simulink model "acc"  (R2018a)
settings: Solver=VariableStepAuto  StartTime=0.0  StopTime=300  FixedStep=0.02  RelTol=1e-3
values from neighbouring files (symbols this model uses):
  b_Ahead = 50    [ACC_DATA.m]    (also in CC_data.m)
  Ctr = 1.6    [ACC_DATA.m]
  F_aero = 1/(2*m_Follower) * Ro_A_Cd    (= 0.000326666666667)    [ACC_DATA.m]
  F_grav = g * sin(theta)    [ACC_DATA.m]
  F_res = Cr * g * cos(theta)    [ACC_DATA.m]
  Kb = 0.005    [ACC_DATA.m]
  Kc = 1    [ACC_DATA.m]
  m_Ahead = 1000    [ACC_DATA.m]    (also in CC_data.m)
  m_Follower = 1500    [ACC_DATA.m]
  r = 0.326    [ACC_DATA.m]
  Rf = 3.28    [ACC_DATA.m]
  Rtr = 1    [ACC_DATA.m]
  Tmax = 528.7 + 0.152*Ne - 0.0000217*Ne^2    (= 789.5)    [ACC_DATA.m]
undefined symbols (not defined in the file or in its folder): sigbuilder_block
libraries: simulink x7
settings Model: Creator=Talha Rao  LastModifiedBy=Talha Rao

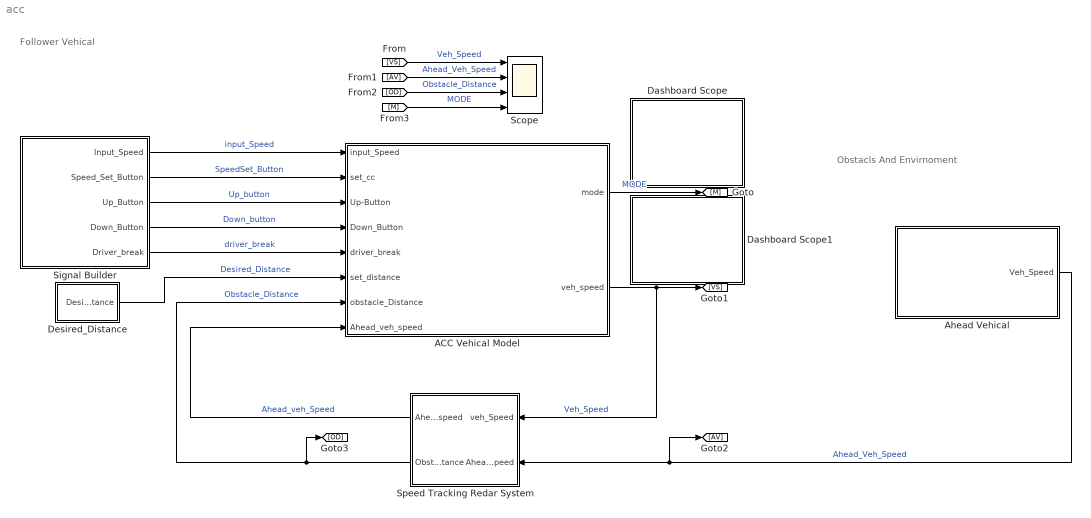
== system acc ==
  note: Follower Vehical
  note: Obstacls And Envirnoment
  ACC Vehical Model : Subsystem
      mask Display: image('C:\Users\Talha Rao\Pictures\carpaint_basic (2).png');
  Ahead Vehical : Subsystem
      mask Display: image('C:\Users\Talha Rao\Pictures\index2 (2).jpg');
  Dashboard Scope : Subsystem  DialogController=hmiCreateDDGDialog  IsWebBlock=on  mask(MWDashboardBlock){webBlockId=e8525703-5d25-447f-a1ea-0cd47b72d774, webBlockType=sdiscope, ShowInitialText=on, HMISrcModelName=acc}
      mask prompts: webBlockId "WebBlock Id"; webBlockType "WebBlock Type"; HMISrcModelName "Source Model"
      mask help: SimulinkHMI:dialogs:HMIScopeDialogDesc
      mask Help: helpview([docroot '/mapfiles/simulink.map'], 'hmi_scope')
      mask Display:
      | if strcmp(get_param(bdroot(gcb),'BlockDiagramType'), 'library')
      |     image([(matlabroot) '/toolbox/simulink/hmi/icons/DashboardScope.png']);
      | end
  Dashboard Scope1 : Subsystem  DialogController=hmiCreateDDGDialog  IsWebBlock=on  mask(MWDashboardBlock){webBlockId=d1b5fd32-8fa1-4132-bafa-763aef0d9398, webBlockType=sdiscope, ShowInitialText=on, HMISrcModelName=acc}
      mask prompts: webBlockId "WebBlock Id"; webBlockType "WebBlock Type"; HMISrcModelName "Source Model"
      mask help: SimulinkHMI:dialogs:HMIScopeDialogDesc
      mask Help: helpview([docroot '/mapfiles/simulink.map'], 'hmi_scope')
      mask Display:
      | if strcmp(get_param(bdroot(gcb),'BlockDiagramType'), 'library')
      |     image([(matlabroot) '/toolbox/simulink/hmi/icons/DashboardScope.png']);
      | end
  Desired_Distance : Subsystem  mask{Desired_Distance=25.0}
      mask DialogControl DescGroupVar Prompt: Set Desired Distance
      mask Display: image('C:\Users\Talha Rao\Pictures\070558928_iconm (2).jpeg');
  Scope : Scope  NumInputPorts=4
  Signal Builder : Subsystem  Tag=STV Subsys  LoadFcn=sigbuilder_block('load',[0 -132 1440 723.6 ]);  StartFcn=sigbuilder_block('start');  StopFcn=sigbuilder_block('stop');  ClipboardFcn=sigbuilder_block('clipboard');  mask(Sigbuilder block){tuvar=[0:10]}
      mask help: Simulink:masks:SigbuilderBlock_MD
      mask init:
      | if ~strcmp(get_param(bdroot(gcbh),'SimulationStatus'),'stopped') tuvar = sigbuilder_block('maskInit'); end
      settings: CopyFcn=sigbuilder_block('copy');  DeleteFcn=sigbuilder_block('delete');  ModelCloseFcn=sigbuilder_block('modelClose');  PreSaveFcn=sigbuilder_block('preSave');  PauseFcn=sigbuilder_block('pause');  ContinueFcn=sigbuilder_block('continue');  NameChangeFcn=sigbuilder_block('namechange');  OpenFcn=sigbuilder_block('open',[0 192 1152 560.25 ]);  CloseFcn=sigbuilder_block('close');
      mask Display: plot(0, 0, 100, 100,[2, 2, 32, 32, 2], [68, 8, 8, 68, 68],[32, 2], [38, 38], [32, 19, 2],[53, 60, 44], [32, 17, 17, 2],[16, 16, 31, 31]);txt = getActiveGroup(gcbh);text(2, 100, txt,'verticalAlignment', 'top');
  Speed Tracking Redar System : Subsystem
      mask Display: image('C:\Users\Talha Rao\Pictures\index3.png');
  wires:
  ACC Vehical Model/2(veh_speed) -> Speed Tracking Redar System/1(veh_Speed), [VS]  "Veh_Speed"
  Speed Tracking Redar System/2(Obstacle_Distance) -> [OD], ACC Vehical Model/7(obstacle_Distance)  "Obstacle_Distance"
  Ahead Vehical/1(Veh_Speed) -> [AV], Speed Tracking Redar System/2(Ahead_Veh_Speed)  "Ahead_Veh_Speed"
  Signal Builder/1(Input_Speed) -> ACC Vehical Model/1(input_Speed)  "input_Speed"
  Signal Builder/3(Up_Button) -> ACC Vehical Model/3(Up-Button)  "Up_button"
  Signal Builder/4(Down_Button) -> ACC Vehical Model/4(Down_Button)  "Down_button"
  Signal Builder/5(Driver_break) -> ACC Vehical Model/5(driver_break)  "driver_break"
  Desired_Distance/1(Desired_Distance) -> ACC Vehical Model/6("set_distance ")  "Desired_Distance"
  Speed Tracking Redar System/1(Ahead_veh_speed) -> ACC Vehical Model/8(Ahead_veh_speed)  "Ahead_veh_Speed"
  [VS] -> Scope/1  "Veh_Speed"
  [AV] -> Scope/2  "Ahead_Veh_Speed"
  [OD] -> Scope/3  "Obstacle_Distance"
  [M] -> Scope/4  "MODE"
  ACC Vehical Model/1(mode) -> [M]  "MODE"
  Signal Builder/2(Speed_Set_Button) -> ACC Vehical Model/2(set_cc)  "SpeedSet_Button"

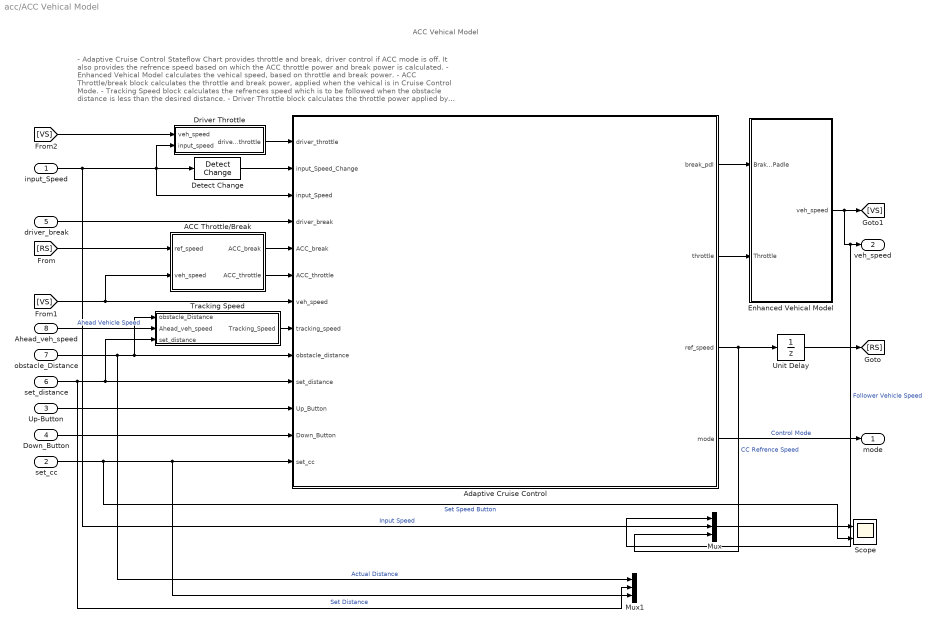
== system acc/ACC Vehical Model ==
  note: - Adaptive Cruise Control Stateflow Chart provides throttle and break, driver control if ACC mode is off. It also provides the refrence speed based on which the ACC throttle power and break power is calculated.
      | - Enhanced Vehical Model calculates the vehical speed, based on throttle and break power.
      | - ACC Throttle/break block calculates the throttle and break power, applied when the vehical is in Cruise Control Mode.
      | - Tracking Speed block calculates the refrences speed which is to be followed when the obstacle distance is less than the desired distance.
      | - Driver Throttle block calculates the throttle power applied by the driver
  note: ACC Vehical Model
  input_Speed : Inport
  set_cc : Inport  Port=2
  Up-Button : Inport  Port=3
  Down_Button : Inport  Port=4
  driver_break : Inport  Port=5
  "set_distance " : Inport  Port=6
  obstacle_Distance : Inport  Port=7
  Ahead_veh_speed : Inport  Port=8
  ACC Throttle/Break : Subsystem
  Adaptive Cruise Control : Stateflow chart  TreatAsAtomicUnit=on
  Detect Change : simulink/Logic and Bit Operations/Detect Change  vinit=0  OutDataTypeStr=boolean
  Driver Throttle : Subsystem
  Enhanced Vehical Model : Subsystem
  Mux : Mux  Inputs=3
  Mux1 : Mux  Inputs=3
  Scope : Scope  NumInputPorts=2
  Tracking Speed : Subsystem
  Unit Delay : UnitDelay  SampleTime=-1
  mode : Outport
  veh_speed : Outport  Port=2
  wires:
  Up-Button/1 -> Adaptive Cruise Control/11(Up_Button)
  Down_Button/1 -> Adaptive Cruise Control/12(Down_Button)
  Detect Change/1 -> Adaptive Cruise Control/2(input_Speed_Change)
  driver_break/1 -> Adaptive Cruise Control/4(driver_break)
  obstacle_Distance/1 -> Mux1/1, Adaptive Cruise Control/9(obstacle_distance), Tracking Speed/1(obstacle_Distance)  "Actual Distance"
  input_Speed/1 -> Mux/2, Adaptive Cruise Control/3(input_Speed), Detect Change/1, Driver Throttle/2(input_speed)  "Input Speed"
  "set_distance "/1 -> Mux1/2, Adaptive Cruise Control/10(set_distance), Tracking Speed/3(set_distance)  "Set Distance"
  ACC Throttle/Break/1(ACC_break) -> Adaptive Cruise Control/5(ACC_break)
  ACC Throttle/Break/2(ACC_throttle) -> Adaptive Cruise Control/6(ACC_throttle)
  [VS] -> Adaptive Cruise Control/7(veh_speed), ACC Throttle/Break/2(veh_speed)
  [RS] -> ACC Throttle/Break/1(ref_speed)
  Adaptive Cruise Control/1(break_pdl) -> Enhanced Vehical Model/1(Brake_Padle)
  Adaptive Cruise Control/2(throttle) -> Enhanced Vehical Model/2(Throttle)
  Enhanced Vehical Model/1(veh_speed) -> Mux/1, veh_speed/1, [VS]  "Follower Vehicle Speed"
  Unit Delay/1 -> [RS]
  Adaptive Cruise Control/4(mode) -> mode/1  "Control Mode"
  Tracking Speed/1(Tracking_Speed) -> Adaptive Cruise Control/8(tracking_speed)
  Ahead_veh_speed/1 -> Tracking Speed/2(Ahead_veh_speed)  "Ahead Vehicle Speed"
  Driver Throttle/1(driver_throttle) -> Adaptive Cruise Control/1(driver_throttle)
  [VS] -> Driver Throttle/1(veh_speed)
  Adaptive Cruise Control/3(ref_speed) -> Mux/3, Unit Delay/1  "CC Refrence Speed"
  set_cc/1 -> Scope/2, Mux1/3, Adaptive Cruise Control/13(set_cc)  "Set Speed Button"
  Mux/1 -> Scope/1

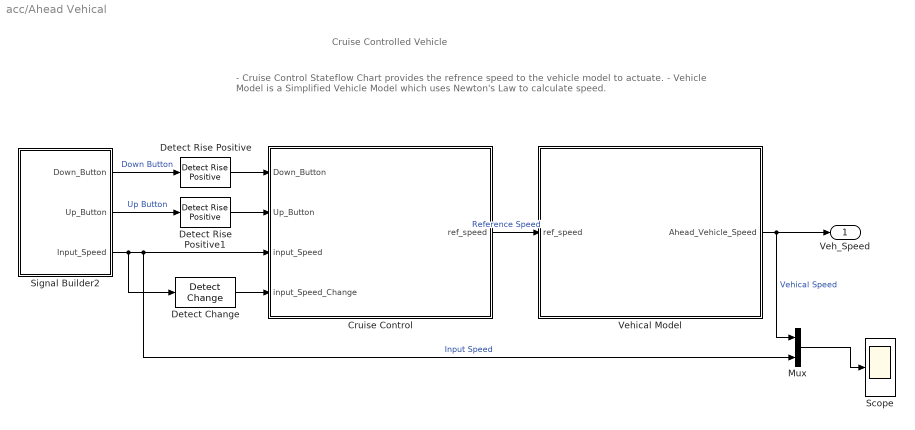
== system acc/Ahead Vehical ==
  note: - Cruise Control Stateflow Chart provides the refrence speed to the vehicle model to actuate.
      | - Vehicle Model is a Simplified Vehicle Model which uses Newton's Law to calculate speed.
  note: Cruise Controlled Vehicle
  Cruise Control : Stateflow chart  TreatAsAtomicUnit=on
  Detect Change : simulink/Logic and Bit Operations/Detect Change  vinit=0  OutDataTypeStr=boolean
  Detect Rise Positive : simulink/Logic and Bit Operations/Detect Rise Positive  vinit=0  OutDataTypeStr=boolean
  Detect Rise Positive1 : simulink/Logic and Bit Operations/Detect Rise Positive  vinit=0  OutDataTypeStr=boolean
  Mux : Mux  Inputs=2
  Scope : Scope
  Signal Builder2 : Subsystem  Tag=STV Subsys  LoadFcn=sigbuilder_block('load');  StartFcn=sigbuilder_block('start');  StopFcn=sigbuilder_block('stop');  ClipboardFcn=sigbuilder_block('clipboard');  mask(Sigbuilder block){tuvar=[0:10]}
      mask help: Simulink:masks:SigbuilderBlock_MD
      mask init:
      | if ~strcmp(get_param(bdroot(gcbh),'SimulationStatus'),'stopped') tuvar = sigbuilder_block('maskInit'); end
      settings: CopyFcn=sigbuilder_block('copy');  DeleteFcn=sigbuilder_block('delete');  ModelCloseFcn=sigbuilder_block('modelClose');  PreSaveFcn=sigbuilder_block('preSave');  PauseFcn=sigbuilder_block('pause');  ContinueFcn=sigbuilder_block('continue');  NameChangeFcn=sigbuilder_block('namechange');  OpenFcn=sigbuilder_block('open',[156 150.75 550.5 399.75 ]);  CloseFcn=sigbuilder_block('close');
      mask Display: plot(0, 0, 100, 100,[2, 2, 32, 32, 2], [68, 8, 8, 68, 68],[32, 2], [38, 38], [32, 19, 2],[53, 60, 44], [32, 17, 17, 2],[16, 16, 31, 31]);txt = getActiveGroup(gcbh);text(2, 100, txt,'verticalAlignment', 'top');
  Vehical Model : Subsystem
  Veh_Speed : Outport
  wires:
  Vehical Model/1(Ahead_Vehicle_Speed) -> Mux/1, Veh_Speed/1  "Vehical Speed"
  Detect Change/1 -> Cruise Control/4(input_Speed_Change)
  Cruise Control/1(ref_speed) -> Vehical Model/1(ref_speed)  "Reference Speed"
  Detect Rise Positive/1 -> Cruise Control/1(Down_Button)
  Signal Builder2/3(Input_Speed) -> Detect Change/1, Mux/2, Cruise Control/3(input_Speed)  "Input Speed"
  Signal Builder2/2(Up_Button) -> Detect Rise Positive1/1  "Up Button"
  Signal Builder2/1(Down_Button) -> Detect Rise Positive/1  "Down Button"
  Detect Rise Positive1/1 -> Cruise Control/2(Up_Button)
  Mux/1 -> Scope/1

== system acc/Dashboard Scope ==

== system acc/Dashboard Scope1 ==

== system acc/Desired_Distance ==
  Constant : Constant  Value=Desired_Distance
  Desired_Distance : Outport
  wires:
  Constant/1 -> Desired_Distance/1

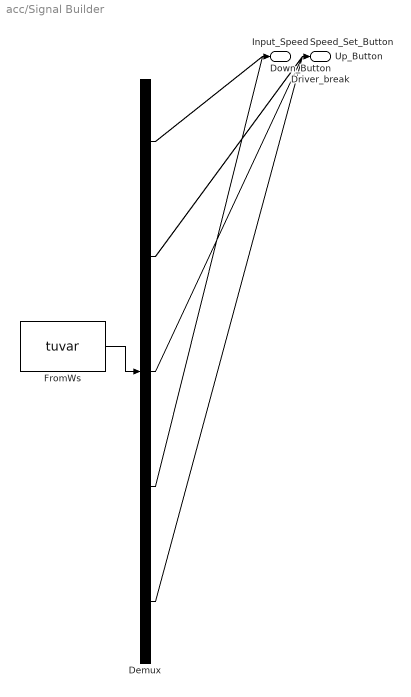
== system acc/Signal Builder ==
  Demux : Demux  Tag=STV Demux  Outputs=5
  FromWs : FromWorkspace  Tag=STV FromWs  VariableName=tuvar  SampleTime=0
      SigBuilderData=|
      | common.afterFinalStr = 'Extrapolate'
      | common.sampleTime = 0
      | dataSet.timeRange = [0 200]
      | dataSet.name = 'Group 1'
      | sbobj.Groups.Name = 'Group 1'
      | sbobj.Groups.Signals(1).Name = 'Input_Speed'
      | sbobj.Groups.Signals(1).XData = [0 12 30 42 43 200]
      | sbobj.Groups.Signals(1).YData = [0 0 112 112 0 0]
      | sbobj.Groups.Signals(2).Name = 'Speed_Set_Button'
      | sbobj.Groups.Signals(2).XData = [0 31 33 200]
      | sbobj.Groups.Signals(2).YData = [0 0 0 0]
      | sbobj.Groups.Signals(3).Name = 'Up_Button'
      | sbobj.Groups.Signals(3).XData = [0 1 200]
      | sbobj.Groups.Signals(3).YData = [0 0 0]
      | sbobj.Groups.Signals(4).Name = 'Down_Button'
      | sbobj.Groups.Signals(4).XData = [0 3 3.4 6 6.4 7 7.4 200]
      | sbobj.Groups.Signals(4).YData = [0 0 0 0 0 0 0 0]
      | sbobj.Groups.Signals(5).Name = 'Driver_break'
      | sbobj.Groups.Signals(5).XData = [0 200]
      | sbobj.Groups.Signals(5).YData = [0 0]
      | sbobj.Groups.TimeRange = [0 200]
  Input_Speed : Outport  Tag=STV Outport
  Speed_Set_Button : Outport  Tag=STV Outport  Port=2
  Up_Button : Outport  Tag=STV Outport  Port=3
  Down_Button : Outport  Tag=STV Outport  Port=4
  Driver_break : Outport  Tag=STV Outport  Port=5
  wires:
  FromWs/1 -> Demux/1
  Demux/1 -> Input_Speed/1
  Demux/2 -> Speed_Set_Button/1
  Demux/3 -> Up_Button/1
  Demux/4 -> Down_Button/1
  Demux/5 -> Driver_break/1

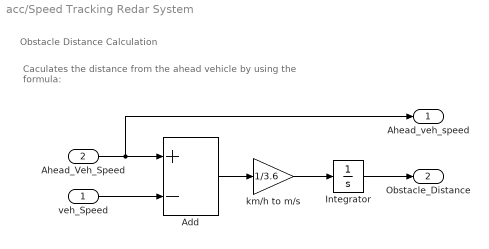
== system acc/Speed Tracking Redar System ==
  note: Caculates the distance from the ahead vehicle by using the formula:
  note: Obstacle Distance Calculation
  veh_Speed : Inport
  Ahead_Veh_Speed : Inport  Port=2
  Add : Sum  Inputs=+-
  Integrator : Integrator  InitialCondition=100
  km/h to m/s : Gain  Gain=1/3.6
  Ahead_veh_speed : Outport
  Obstacle_Distance : Outport  Port=2
  wires:
  Ahead_Veh_Speed/1 -> Ahead_veh_speed/1, Add/1
  veh_Speed/1 -> Add/2
  Add/1 -> km/h to m/s/1
  km/h to m/s/1 -> Integrator/1
  Integrator/1 -> Obstacle_Distance/1

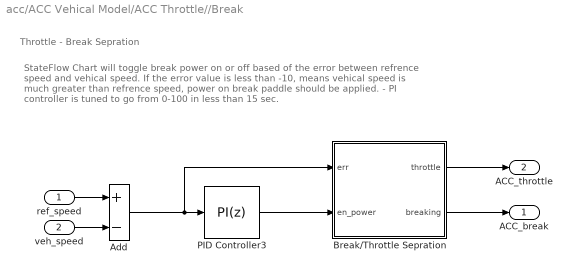
== system acc/ACC Vehical Model/ACC Throttle//Break ==
  note: StateFlow Chart will toggle break power on or off based of the error between refrence speed and
      | vehical speed. If the error value is less than -10, means vehical speed is much greater than refrence
      | speed, power on break paddle should be applied.
      |
      | - PI controller is tuned to go from 0-100 in less than 15 sec.
  note: Throttle - Break Sepration
  ref_speed : Inport
  veh_speed : Inport  Port=2
  Add : Sum  Inputs=+-
  Break/Throttle Sepration : Stateflow chart  TreatAsAtomicUnit=on
  PID Controller3 : simulink/Continuous/PID Controller  Controller=PI  TimeDomain=Discrete-time  SampleTime=0.02  IntegratorMethod=Trapezoidal  FilterMethod=Forward Euler  Form=Parallel  UseFilter=on  ControllerParametersSource=internal  P=5  I=0.5  D=0  N=100  InitialConditionSource=internal  InitialConditionForIntegrator=0  InitialConditionForFilter=0  ExternalReset=none  LimitOutput=on  UpperSaturationLimit=100  LowerSaturationLimit=-100  LinearizeAsGain=on  AntiWindupMode=clamping  Kb=1  TrackingMode=off  Kt=1  PParamMin=[]  PParamMax=[]  IParamMin=[]  IParamMax=[]  DParamMin=[]  DParamMax=[]  NParamMin=[]  NParamMax=[]  KbParamMin=[]  KbParamMax=[]  KtParamMin=[]  KtParamMax=[]  POutMin=[]  POutMax=[]  IOutMin=[]  IOutMax=[]  DOutMin=[]  DOutMax=[]  NOutMin=[]  NOutMax=[]  KbOutMin=[]  KbOutMax=[]  KtOutMin=[]  KtOutMax=[]  IntegratorOutMin=[]  IntegratorOutMax=[]  FilterOutMin=[]  FilterOutMax=[]  SumOutMin=[]  SumOutMax=[]  SumI1OutMin=[]  SumI1OutMax=[]  SumI2OutMin=[]  SumI2OutMax=[]  SumI3OutMin=[]  SumI3OutMax=[]  SumDOutMin=[]  SumDOutMax=[]  SaturationOutMin=[]  SaturationOutMax=[]  IntegratorContinuousStateAttributes=''  IntegratorStateMustResolveToSignalObject=off  IntegratorRTWStateStorageClass=Auto  FilterContinuousStateAttributes=''  FilterStateMustResolveToSignalObject=off  FilterRTWStateStorageClass=Auto  DifferentiatorICPrevScaledInput=0  DifferentiatorOutMin=[]  DifferentiatorOutMax=[]  FilterDiffOutCoefMin=[]  FilterDiffOutCoefMax=[]  SumDenOutMin=[]  SumDenOutMax=[]  SumNumOutMin=[]  SumNumOutMax=[]  ReciprocalOutMin=[]  ReciprocalOutMax=[]  DivideOutMin=[]  DivideOutMax=[]  TunerSelectOption=Transfer Function Based (PID Tuner App)
  ACC_break : Outport
  ACC_throttle : Outport  Port=2
  wires:
  ref_speed/1 -> Add/1
  veh_speed/1 -> Add/2
  Break/Throttle Sepration/1(throttle) -> ACC_throttle/1
  Break/Throttle Sepration/2(breaking) -> ACC_break/1
  PID Controller3/1 -> Break/Throttle Sepration/2(en_power)
  Add/1 -> Break/Throttle Sepration/1(err), PID Controller3/1

== system acc/ACC Vehical Model/Driver Throttle ==
  note: This block calculates the throttle power needs to be applied in order to attain the input speed
      | - PI controller is tuned to go from 0-100 in less than 15 sec.
  note: Driver Throttle
  veh_speed : Inport
  input_speed : Inport  Port=2
  Add : Sum  Inputs=+-
  PID Controller3 : simulink/Continuous/PID Controller  Controller=PI  TimeDomain=Discrete-time  SampleTime=0.02  IntegratorMethod=Trapezoidal  FilterMethod=Forward Euler  Form=Parallel  UseFilter=on  ControllerParametersSource=internal  P=5  I=0.5  D=0  N=100  InitialConditionSource=internal  InitialConditionForIntegrator=0  InitialConditionForFilter=0  ExternalReset=none  LimitOutput=on  UpperSaturationLimit=100  LowerSaturationLimit=-100  LinearizeAsGain=on  AntiWindupMode=clamping  Kb=1  TrackingMode=off  Kt=1  PParamMin=[]  PParamMax=[]  IParamMin=[]  IParamMax=[]  DParamMin=[]  DParamMax=[]  NParamMin=[]  NParamMax=[]  KbParamMin=[]  KbParamMax=[]  KtParamMin=[]  KtParamMax=[]  POutMin=[]  POutMax=[]  IOutMin=[]  IOutMax=[]  DOutMin=[]  DOutMax=[]  NOutMin=[]  NOutMax=[]  KbOutMin=[]  KbOutMax=[]  KtOutMin=[]  KtOutMax=[]  IntegratorOutMin=[]  IntegratorOutMax=[]  FilterOutMin=[]  FilterOutMax=[]  SumOutMin=[]  SumOutMax=[]  SumI1OutMin=[]  SumI1OutMax=[]  SumI2OutMin=[]  SumI2OutMax=[]  SumI3OutMin=[]  SumI3OutMax=[]  SumDOutMin=[]  SumDOutMax=[]  SaturationOutMin=[]  SaturationOutMax=[]  IntegratorContinuousStateAttributes=''  IntegratorStateMustResolveToSignalObject=off  IntegratorRTWStateStorageClass=Auto  FilterContinuousStateAttributes=''  FilterStateMustResolveToSignalObject=off  FilterRTWStateStorageClass=Auto  DifferentiatorICPrevScaledInput=0  DifferentiatorOutMin=[]  DifferentiatorOutMax=[]  FilterDiffOutCoefMin=[]  FilterDiffOutCoefMax=[]  SumDenOutMin=[]  SumDenOutMax=[]  SumNumOutMin=[]  SumNumOutMax=[]  ReciprocalOutMin=[]  ReciprocalOutMax=[]  DivideOutMin=[]  DivideOutMax=[]  TunerSelectOption=Transfer Function Based (PID Tuner App)
  driver_throttle : Outport
  wires:
  input_speed/1 -> Add/1
  veh_speed/1 -> Add/2
  PID Controller3/1 -> driver_throttle/1
  Add/1 -> PID Controller3/1

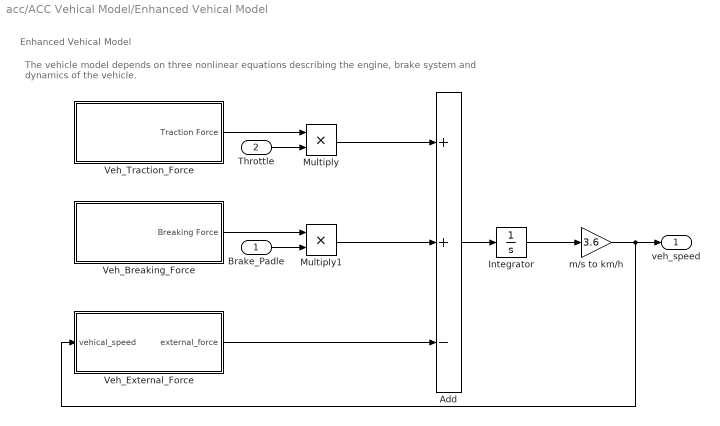
== system acc/ACC Vehical Model/Enhanced Vehical Model ==
  note: The vehicle model depends on three nonlinear equations describing the engine, brake system and dynamics of the vehicle.
  note: Enhanced Vehical Model
  Brake_Padle : Inport
  Throttle : Inport  Port=2
  Add : Sum  Inputs=++-
  Integrator : Integrator
  Multiply : Product
  Multiply1 : Product
  Veh_Breaking_Force : Subsystem
  Veh_External_Force : Subsystem
  Veh_Traction_Force : Subsystem
  m/s to km/h : Gain  Gain=3.6
  veh_speed : Outport
  wires:
  Veh_External_Force/1(external_force) -> Add/3
  Brake_Padle/1 -> Multiply1/2
  Veh_Breaking_Force/1("Breaking Force ") -> Multiply1/1
  Throttle/1 -> Multiply/2
  Multiply1/1 -> Add/2
  Multiply/1 -> Add/1
  Veh_Traction_Force/1(Traction Force) -> Multiply/1
  Add/1 -> Integrator/1
  Integrator/1 -> m/s to km/h/1
  m/s to km/h/1 -> Veh_External_Force/1(vehical_speed), veh_speed/1

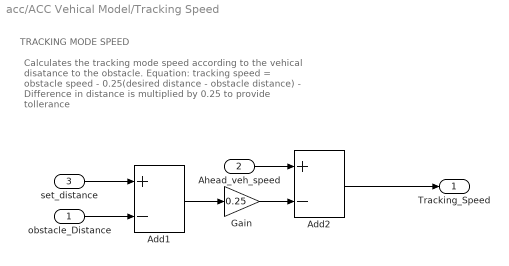
== system acc/ACC Vehical Model/Tracking Speed ==
  note: Calculates the tracking mode speed according to the vehical disatance
      | to the obstacle.
      | Equation:
      |
      | tracking speed = obstacle speed - 0.25(desired distance - obstacle distance)
      |
      | - Difference in distance is multiplied by 0.25 to provide tollerance
  note: TRACKING MODE SPEED
  obstacle_Distance : Inport
  Ahead_veh_speed : Inport  Port=2
  set_distance : Inport  Port=3
  Add1 : Sum  Inputs=+-
  Add2 : Sum  Inputs=+-
  Gain : Gain  Gain=0.25
  Tracking_Speed : Outport
  wires:
  Add1/1 -> Gain/1
  Gain/1 -> Add2/2
  Ahead_veh_speed/1 -> Add2/1
  Add2/1 -> Tracking_Speed/1
  set_distance/1 -> Add1/1
  obstacle_Distance/1 -> Add1/2

== system acc/Ahead Vehical/Signal Builder2 ==
  Demux : Demux  Tag=STV Demux  Outputs=3
  FromWs : FromWorkspace  Tag=STV FromWs  VariableName=tuvar  SampleTime=0
      SigBuilderData=|
      | common.afterFinalStr = 'Extrapolate'
      | common.sampleTime = 0
      | dataSet.timeRange = [0 200]
      | dataSet.name = 'Group 1'
      | sbobj.Groups.Name = 'Group 1'
      | sbobj.Groups.Signals(1).Name = 'Down_Button'
      | sbobj.Groups.Signals(1).XData = [0 200]
      | sbobj.Groups.Signals(1).YData = [0 0]
      | sbobj.Groups.Signals(2).Name = 'Up_Button'
      | sbobj.Groups.Signals(2).XData = [0 1 200]
      | sbobj.Groups.Signals(2).YData = [0 0 0]
      | sbobj.Groups.Signals(3).Name = 'Input_Speed'
      | sbobj.Groups.Signals(3).XData = [0 5 25 38 80 120 140 175 195 200]
      | sbobj.Groups.Signals(3).YData = [0 0 100 100 98 98 115 115 94 94]
      | sbobj.Groups.TimeRange = [0 200]
  Down_Button : Outport  Tag=STV Outport
  Up_Button : Outport  Tag=STV Outport  Port=2
  Input_Speed : Outport  Tag=STV Outport  Port=3
  wires:
  FromWs/1 -> Demux/1
  Demux/1 -> Down_Button/1
  Demux/2 -> Up_Button/1
  Demux/3 -> Input_Speed/1

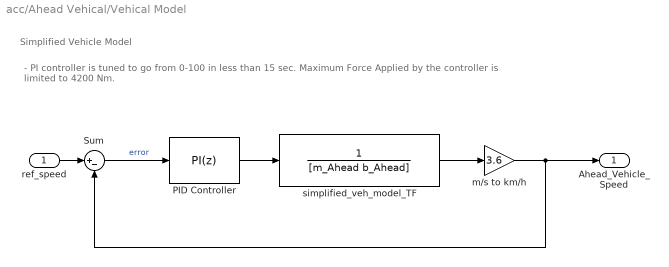
== system acc/Ahead Vehical/Vehical Model ==
  note: Simplified Vehicle Model
  note: - PI controller is tuned to go from 0-100 in less than 15 sec. Maximum Force Applied by the controller is limited to 4200 Nm.
  ref_speed : Inport
  PID Controller : simulink/Continuous/PID Controller  Controller=PI  TimeDomain=Discrete-time  SampleTime=0.001  IntegratorMethod=Forward Euler  FilterMethod=Forward Euler  Form=Parallel  UseFilter=on  ControllerParametersSource=internal  P=125  I=7.2  D=0.02  N=20  InitialConditionSource=internal  InitialConditionForIntegrator=0  InitialConditionForFilter=0  ExternalReset=none  LimitOutput=on  UpperSaturationLimit=4200  LowerSaturationLimit=0  LinearizeAsGain=on  AntiWindupMode=none  Kb=1  TrackingMode=off  Kt=1  PParamMin=[]  PParamMax=[]  IParamMin=[]  IParamMax=[]  DParamMin=[]  DParamMax=[]  NParamMin=[]  NParamMax=[]  KbParamMin=[]  KbParamMax=[]  KtParamMin=[]  KtParamMax=[]  POutMin=[]  POutMax=[]  IOutMin=[]  IOutMax=[]  DOutMin=[]  DOutMax=[]  NOutMin=[]  NOutMax=[]  KbOutMin=[]  KbOutMax=[]  KtOutMin=[]  KtOutMax=[]  IntegratorOutMin=[]  IntegratorOutMax=[]  FilterOutMin=[]  FilterOutMax=[]  SumOutMin=[]  SumOutMax=[]  SumI1OutMin=[]  SumI1OutMax=[]  SumI2OutMin=[]  SumI2OutMax=[]  SumI3OutMin=[]  SumI3OutMax=[]  SumDOutMin=[]  SumDOutMax=[]  SaturationOutMin=[]  SaturationOutMax=[]  IntegratorContinuousStateAttributes=''  IntegratorStateMustResolveToSignalObject=off  IntegratorRTWStateStorageClass=Auto  FilterContinuousStateAttributes=''  FilterStateMustResolveToSignalObject=off  FilterRTWStateStorageClass=Auto  DifferentiatorICPrevScaledInput=0  DifferentiatorOutMin=[]  DifferentiatorOutMax=[]  FilterDiffOutCoefMin=[]  FilterDiffOutCoefMax=[]  SumDenOutMin=[]  SumDenOutMax=[]  SumNumOutMin=[]  SumNumOutMax=[]  ReciprocalOutMin=[]  ReciprocalOutMax=[]  DivideOutMin=[]  DivideOutMax=[]  TunerSelectOption=Transfer Function Based (PID Tuner App)
  Sum : Sum  Inputs=|+-
  m/s to km/h : Gain  Gain=3.6
  simplified_veh_model_TF : TransferFcn  Denominator=[m_Ahead b_Ahead]
  Ahead_Vehicle_Speed : Outport
  wires:
  ref_speed/1 -> Sum/1
  Sum/1 -> PID Controller/1  "error"
  m/s to km/h/1 -> Sum/2, Ahead_Vehicle_Speed/1
  simplified_veh_model_TF/1 -> m/s to km/h/1
  PID Controller/1 -> simplified_veh_model_TF/1

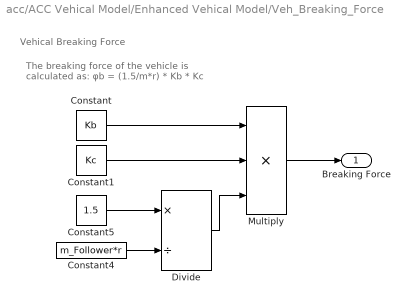
== system acc/ACC Vehical Model/Enhanced Vehical Model/Veh_Breaking_Force ==
  note: Vehical Breaking Force
  note: The breaking force of the vehicle is calculated as:
      | φb = (1.5/m*r) * Kb * Kc
  Constant : Constant  Value=Kb
  Constant1 : Constant  Value=Kc
  Constant4 : Constant  Value=m_Follower*r
  Constant5 : Constant  Value=1.5
  Divide : Product  Inputs=*/
  Multiply : Product  Inputs=3
  "Breaking Force " : Outport
  wires:
  Multiply/1 -> "Breaking Force "/1
  Constant4/1 -> Divide/2
  Constant1/1 -> Multiply/2
  Constant/1 -> Multiply/1
  Constant5/1 -> Divide/1
  Divide/1 -> Multiply/3

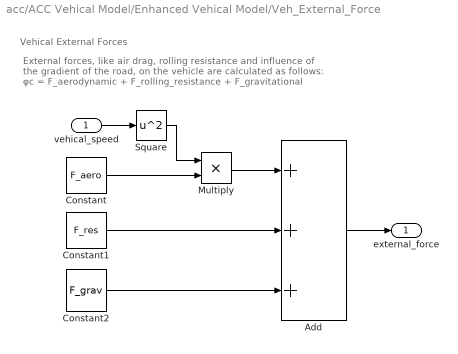
== system acc/ACC Vehical Model/Enhanced Vehical Model/Veh_External_Force ==
  note: External forces, like air drag, rolling resistance and
      | influence of the gradient of the road, on the vehicle are calculated as follows:
      |
      | φc = F_aerodynamic + F_rolling_resistance + F_gravitational
  note: Vehical External Forces
  vehical_speed : Inport
  Add : Sum  Inputs=+++
  Constant : Constant  Value=F_aero
  Constant1 : Constant  Value=F_res
  Constant2 : Constant  Value=F_grav
  Multiply : Product
  Square : Math  Operator=square  SaturateOnIntegerOverflow=on
  external_force : Outport
  wires:
  Add/1 -> external_force/1
  Constant1/1 -> Add/2
  Constant2/1 -> Add/3
  Constant/1 -> Multiply/2
  vehical_speed/1 -> Square/1
  Square/1 -> Multiply/1
  Multiply/1 -> Add/1

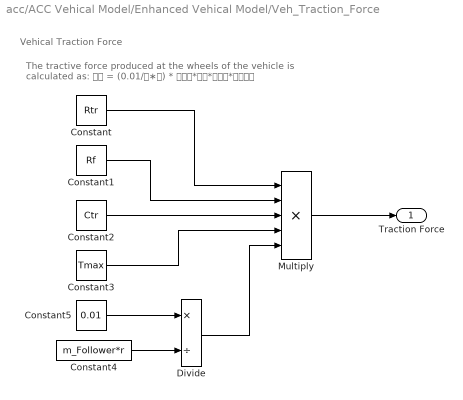
== system acc/ACC Vehical Model/Enhanced Vehical Model/Veh_Traction_Force ==
  note: The tractive force produced at the wheels of the vehicle is calculated as:
      | 𝜑𝑡 = (0.01/𝑚∗𝑟) * 𝑅𝑡𝑟*𝑅𝑓*𝐶𝑡𝑟*𝑇𝑚𝑎𝑥
  note: Vehical Traction Force
  Constant : Constant  Value=Rtr
  Constant1 : Constant  Value=Rf
  Constant2 : Constant  Value=Ctr
  Constant3 : Constant  Value=Tmax
  Constant4 : Constant  Value=m_Follower*r
  Constant5 : Constant  Value=0.01
  Divide : Product  Inputs=*/
  Multiply : Product  Inputs=5
  Traction Force : Outport
  wires:
  Constant/1 -> Multiply/1
  Constant4/1 -> Divide/2
  Constant1/1 -> Multiply/2
  Constant5/1 -> Divide/1
  Constant3/1 -> Multiply/4
  Divide/1 -> Multiply/5
  Constant2/1 -> Multiply/3
  Multiply/1 -> Traction Force/1

== stateflow chart acc/ACC Vehical Model/ACC Throttle//Break/Break//Throttle Sepration ==
  note: Break/Throttle Separation
  note: State
      | Description
      | Condition
      | Next State
      |
      | OPEN_THROTTLE
      | Apply power on throttle when error is >= -10
      | err >= -10
      | APPLY_BREAK
      |
      | APPLY_BREAK
      | Apply power on break when error is < -10
      | err < -10
      | OPEN_THROTTLE
  state OPEN_THROTTLE
    en: breaking = 0;
    during: throttle = en_power;
  state APPLY_BREAK
    during: breaking = en_power;
    en:throttle = 0;
  (default) -> OPEN_THROTTLE
  OPEN_THROTTLE -> APPLY_BREAK : [err<-5]
  APPLY_BREAK -> OPEN_THROTTLE : [err >= 0]
  data: throttle output; breaking output; err input; en_power input

== stateflow chart acc/Ahead Vehical/Cruise Control ==
  note: Cruise Control
  note: State
      | Description
      | Condition
      | Next State
      |
      | CRUISE_ONTROL_ON
      | Default State where ref_speed is initially set to input speed
      | Default
      | UP_BUTTON_PRESSED / DOWN_BUTTON_PRESSED /
      | REFRESH_TO_REFRENCE
      |
      | UP_BUTTON_PRESSED
      | If the up button is pressed, increase speed by 5 km/h and return to default state immediately.
      | UP_BUTTON is pressed
      | CRUISE_ONTROL_ON
      |
      | DOWN_BUTTON_PRESSED
      | If the down button is pressed, decrease speed by 5 km/h and return to default state immediately.
      | DOWN_BUTTON is pressed
      | CRUISE_ONTROL_ON
      |
      | REFRESH_TO_REFRENCE
      | If system detects a change in input speed, overrule the previous refrence speed and adjust to the new input speed. Leaves the state if refrence speed becomes equal to input speed
      | Input Speed is changed
      | CRUISE_ONTROL_ON
  state UP_BUTTON_PRESSED
    ref_speed = ref_speed + 5;
  state DOWN_BUTTON_PRESSED
    ref_speed = ref_speed - 5;
  state CRUISE_ONTROL_ON
    ref_speed = ref_speed;
  state REFRESH_TO_REFRENCE
    ref_speed = input_Speed;
  (default) -> CRUISE_ONTROL_ON : {ref_speed = input_Speed}
  CRUISE_ONTROL_ON -> DOWN_BUTTON_PRESSED [order 2] : [Down_Button>0]
  CRUISE_ONTROL_ON -> UP_BUTTON_PRESSED [order 1] : [Up_Button > 0]
  DOWN_BUTTON_PRESSED -> CRUISE_ONTROL_ON
  UP_BUTTON_PRESSED -> CRUISE_ONTROL_ON
  REFRESH_TO_REFRENCE -> CRUISE_ONTROL_ON : [input_Speed == ref_speed]
  CRUISE_ONTROL_ON -> REFRESH_TO_REFRENCE [order 3] : [input_Speed_Change > 0]
  data: Down_Button input; Up_Button input; input_Speed input; input_Speed_Change input; ref_speed output

== stateflow chart acc/ACC Vehical Model/Adaptive Cruise Control ==
  settings: executeAtInitialization=1
  note: Adaptive Cruise Control
  note: ACC LOGIC
  note: ACTUATOR LOGIC
  note: State
      | Description
      | Condition
      | Next State
      |
      | IDLE_STATE
      | Set cc refrence speed & set_speed equal to input speed
      | default || ACC_OFF
      | SPEED_TRACKING
      |
      | SPEED_TRACKING
      | Follow the set speed chosen by the driver
      | ACC_ON event occured && obstacle_distance < set_distance
      | DISTANCE_TRACKING / IDLE_STATE
      |
      | DISTANCE_TRACKING
      | Follow the tracking speed to keep the min distance maintained
      | obstacle_distance > set_distance...
      | && after(60,sec)
      | SPEED_TRACKING
  note: State
      | Description
      | Condition
      | Next State
      |
      | ACC_OFF
      | Generate ACC_OFF event upon entry. Set throttle and break to Driver throttle and break.
      | default / break paddle is pressed
      | ACC_ON
      |
      | ACC_ON
      | Set throttle and break to ACC throttle and ACC break. Generate ACC_ON event upon entry. Keep track of the set speed button.
      | veh_speed>30
      | ACC_OFF
  state ACC_LOGIC [parallel]
    settings: executionOrder=2
    state SPEED_TRACKING
      mode = speedTracking;
      state UP_BUTTON_PRESSED
        ref_speed = ref_speed + 5;
      state DOWN_BUTTON_PRESSED
        ref_speed = ref_speed - 5;
      state Cruise_Control_ON
        en: ref_speed = set_speed;
        ref_speed = ref_speed;
      state REFRESH_TO_REFRENCE
        ref_speed = input_Speed;
        exit: set_speed = input_Speed;
      (default) -> Cruise_Control_ON
      Cruise_Control_ON -> DOWN_BUTTON_PRESSED [order 2] : [Down_Button>0]
      Cruise_Control_ON -> UP_BUTTON_PRESSED [order 1] : [Up_Button > 0]
      DOWN_BUTTON_PRESSED -> Cruise_Control_ON
      UP_BUTTON_PRESSED -> Cruise_Control_ON
      REFRESH_TO_REFRENCE -> Cruise_Control_ON : [(input_Speed == ref_speed...
          |  && after (30,sec) )...
          |  || ss_button > 0]
      Cruise_Control_ON -> REFRESH_TO_REFRENCE [order 3] : [input_Speed_Change > 0 ...
          |  && ss_button ==0 ]
    state IDLE_STATE
      ref_speed = ...
      input_Speed;
      set_speed =...
      input_Speed;
    state DISTANCE_TRACKING
      ref_speed = tracking_speed;
      mode =distanceTracking;
    (default) -> IDLE_STATE
    IDLE_STATE -> SPEED_TRACKING : ACC_ON
    SPEED_TRACKING -> IDLE_STATE [order 2] : ACC_OFF
    DISTANCE_TRACKING -> SPEED_TRACKING : [obstacle_distance > set_distance...
        | && after(60,sec) ]
    SPEED_TRACKING -> DISTANCE_TRACKING [order 1] : [obstacle_distance...
        | < set_distance]
  state ACTUATOR_LOGIC [parallel]
    settings: executionOrder=1
    state ACC_OFF
      send(ACC_OFF, ACC_LOGIC);
      throttle = driver_throttle;
      break_pdl = driver_break;
      mode =driverControl;
    state ACC_ON
      en: ss_button = false;
      en: send(ACC_ON, ACC_LOGIC);
      du: throttle = ACC_throttle;
      du: break_pdl = ACC_break;
      state SS_BUTTON_UNPRESSED
        en: ss_button = false;
      state SS_BUTTON_PRESSED
        en: ss_button = true;
        en: set_speed = input_Speed;
      (default) -> SS_BUTTON_UNPRESSED
      SS_BUTTON_UNPRESSED -> SS_BUTTON_PRESSED : [set_cc>0]
    (default) -> ACC_OFF
    ACC_OFF -> ACC_ON : [veh_speed>30]
    ACC_ON -> ACC_OFF : [driver_break>0]
  data: driver_throttle input; input_Speed_Change input; input_Speed input; driver_break input; ACC_break input; ACC_throttle input; veh_speed input; tracking_speed input; obstacle_distance input; set_distance input; Up_Button input; Down_Button input; set_cc input; break_pdl output; throttle output; ref_speed output; st local boolean; sp local boolean; mode output Enum: control_mode_type; set_speed local; ss_button local boolean
  events: set_button local FUNCTION_CALL_EVENT; ACC_ON local RISING_EDGE_EVENT; ACC_OFF local RISING_EDGE_EVENT
